simulink model "ColourTesting02_16_23"  (R2022a)
settings: Solver=VariableStepAuto  StartTime=0.0  StopTime=inf  RelTol=1e-3
model workspace (MAT data in the model file):
  SL_ROS_VariableLengthArrays_MaxSizes.CommonInfo.ArrayTruncateAction = 'EmitWarning'
  SL_ROS_VariableLengthArrays_MaxSizes.MsgTypeMap = containers.Map
  SL_ROS_VariableLengthArrays_MaxSizes.MsgTypeMap.serialization.keys = {'sensor_msgs/Image'}
  SL_ROS_VariableLengthArrays_MaxSizes.MsgTypeMap.serialization.values{1}(1).PropertyName = 'Data'
  SL_ROS_VariableLengthArrays_MaxSizes.MsgTypeMap.serialization.values{1}(1).DataType = 'uint8'
  SL_ROS_VariableLengthArrays_MaxSizes.MsgTypeMap.serialization.values{1}(1).MaxLength = 3686400
  SL_ROS_VariableLengthArrays_MaxSizes.MsgTypeMap.serialization.values{1}(2).PropertyName = 'Encoding'
  SL_ROS_VariableLengthArrays_MaxSizes.MsgTypeMap.serialization.values{1}(2).DataType = 'uint8'
  SL_ROS_VariableLengthArrays_MaxSizes.MsgTypeMap.serialization.values{1}(2).MaxLength = 128
  SL_ROS_VariableLengthArrays_MaxSizes.MsgTypeMap.serialization.uniformity = 0
  SL_ROS_VariableLengthArrays_MaxSizes.MsgTypeMap.serialization.keyType = 'char'
  SL_ROS_VariableLengthArrays_MaxSizes.MsgTypeMap.serialization.valueType = 'any'
undefined symbols (not defined in the file): coder, ros
libraries: robotlib x13
settings Model: SimulationMode=accelerator  Creator=ll  LastModifiedBy=ll

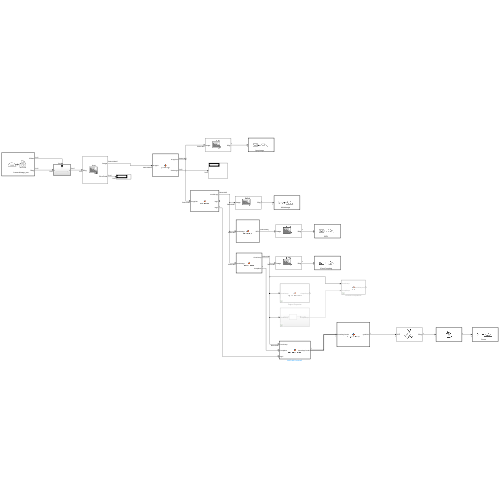
[thumbnail: Simulink's stored preview of the top-level diagram]
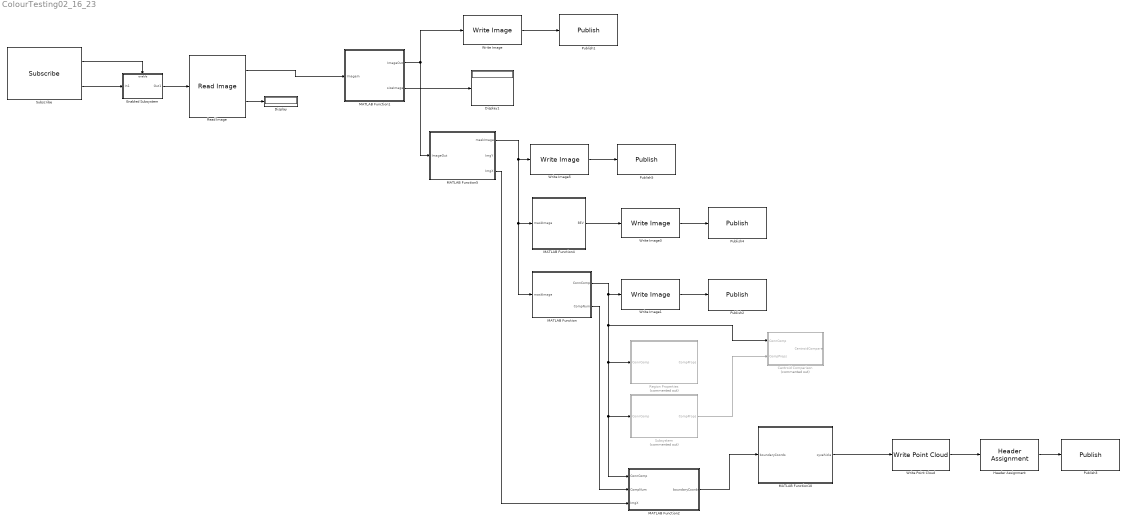
== system ColourTesting02_16_23 ==
  Centroid Comparison : MATLAB Function  Commented=on  TreatAsAtomicUnit=on
  Display : Display
  Display1 : Display
  Enabled Subsystem : Subsystem  TreatAsAtomicUnit=on
  Header Assignment : robotlib/Header Assignment  SetFrameID=on  FrameID=map  InsertTimeStamp=on  SetHeaderFieldName=Use the default Header field name  HeaderFieldName=Header
      settings: SourceProductBaseCode=RR
  MATLAB Function : MATLAB Function  TreatAsAtomicUnit=on
  MATLAB Function1 : MATLAB Function  TreatAsAtomicUnit=on
  MATLAB Function10 : MATLAB Function  TreatAsAtomicUnit=on
  MATLAB Function2 : MATLAB Function  TreatAsAtomicUnit=on
  MATLAB Function4 : MATLAB Function  TreatAsAtomicUnit=on
  MATLAB Function5 : MATLAB Function  TreatAsAtomicUnit=on
  Publish1 : robotlib/Publish  topicSource=Specify your own  topic=/grayimage  messageType=sensor_msgs/Image  legacyBusStruct=off  messageQueueLength=1
  Publish2 : robotlib/Publish  topicSource=Specify your own  topic=/ConnCompImg  messageType=sensor_msgs/Image  legacyBusStruct=off  messageQueueLength=1
  Publish3 : robotlib/Publish  topicSource=Specify your own  topic=/lanes  messageType=sensor_msgs/PointCloud2  legacyBusStruct=off  messageQueueLength=1
  Publish4 : robotlib/Publish  topicSource=Specify your own  topic=/BEV  messageType=sensor_msgs/Image  legacyBusStruct=off  messageQueueLength=1
  Publish5 : robotlib/Publish  topicSource=Specify your own  topic=/whiteimage  messageType=sensor_msgs/Image  legacyBusStruct=off  messageQueueLength=1
  Read Image : robotlib/Read Image  MaximumImageSize=[960, 1280]  ImageEncoding=bgr8  ShowAlphaOutput=off  ShowErrorCodeOutput=on  VariableSizeOutputs=off
      settings: SourceProductBaseCode=RR
  Region Properties : MATLAB Function  Commented=on  TreatAsAtomicUnit=on
  Subscribe : robotlib/Subscribe  topicSource=Select from ROS network  topic=/camera/image_raw  messageType=sensor_msgs/Image  SampleTime=-1  legacyBusStruct=off  messageQueueLength=1
  Subsystem : Subsystem  Commented=on
  Write Image{,1,3,5} (4 alike) : robotlib/Write Image  ImageEncoding=mono8  EncodingStruct=ros.msg.sensor_msgs.internal.ImageEncoding.info(coder.const('mono8'))  HasAlpha=off  messageType=sensor_msgs/Image
      settings: SourceProductBaseCode=RR
  Write Point Cloud : robotlib/Write Point Cloud  Encoding=none  HasRGB=false  HasAlpha=false  FieldNamesStruct=struct('x', 'single', 'y', 'single', 'z', 'single')  messageType=sensor_msgs/PointCloud2
      settings: SourceProductBaseCode=RR
  wires:
  Subscribe/2 -> Enabled Subsystem/1(In1)
  Enabled Subsystem/1(Out1) -> Read Image/1
  Subscribe/1 -> Enabled Subsystem/Enable
  Read Image/2 -> Display/1
  Read Image/1 -> MATLAB Function1/1(ImageIn)
  Write Image/1 -> Publish1/1
  MATLAB Function1/1(ImageOut) -> MATLAB Function5/1(ImageOut), Write Image/1
  MATLAB Function1/2(sizeImage) -> Display1/1
  MATLAB Function5/1(maskImage) -> MATLAB Function4/1(maskImage), MATLAB Function/1(maskImage), Write Image5/1
  Write Image5/1 -> Publish5/1
  MATLAB Function4/1(BEV) -> Write Image3/1
  Write Image3/1 -> Publish4/1
  MATLAB Function/1(ConnComp) -> Centroid Comparison/1(ConnComp), MATLAB Function2/1(ConnComp), Subsystem/1(ConnComp), Region Properties/1(ConnComp), Write Image1/1
  Write Image1/1 -> Publish2/1
  Subsystem/1(CompProps) -> Centroid Comparison/2(CompProps)
  MATLAB Function2/1(boundaryCoords) -> MATLAB Function10/1(boundaryCoords)
  MATLAB Function/2(CompNum) -> MATLAB Function2/2(CompNum)
  MATLAB Function5/3(ImgX) -> MATLAB Function2/3(ImgX)
  Header Assignment/1 -> Publish3/1
  Write Point Cloud/1 -> Header Assignment/1
  MATLAB Function10/1(xyvehicle) -> Write Point Cloud/1

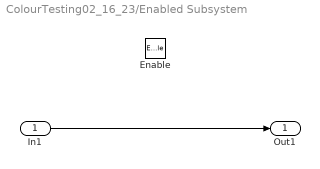
== system ColourTesting02_16_23/Enabled Subsystem ==
  In1 : Inport
  Enable : EnablePort
  Out1 : Outport
  wires:
  In1/1 -> Out1/1

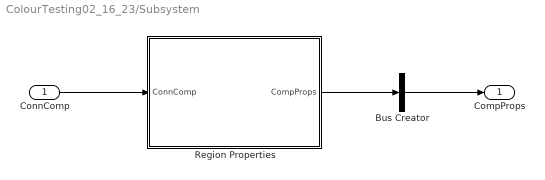
== system ColourTesting02_16_23/Subsystem ==
  ConnComp : Inport
  Bus Creator : BusCreator  Inputs=1
  Region Properties : MATLAB Function  TreatAsAtomicUnit=on
  CompProps : Outport
  wires:
  ConnComp/1 -> Region Properties/1(ConnComp)
  Region Properties/1(CompProps) -> Bus Creator/1
  Bus Creator/1 -> CompProps/1

== matlab function ColourTesting02_16_23/MATLAB Function1 ==
  data: ImageIn input; ImageOut output; sizeImage output
function [ImageOut,sizeImage] = grayImage(ImageIn)

sizeImage=size(ImageIn);

ImageOut=im2uint8(im2gray(ImageIn));

== matlab function ColourTesting02_16_23/MATLAB Function4 ==
  data: maskImage input; BEV output
function BEV = BEVimage(maskImage)
%Transform Road Image to Bird's-Eye-View Image
%Create a bird's-eye-view image from an image obtained by a front-facing 
% camera mounted on a vehicle. Display points within the bird's-eye view 
% using the vehicle and image coordinate systems.
%Define the camera intrinsics and create an object containing these intrinsics.
%focalLength = [309.4362 344.2161];
%focalLength=[274.769879268627	124.585825090253];
focalLength=[9.485122935354788e+02,9.419404214092846e+02];
%249.386359893401	113.313356588451
%principalPoint = [318.9034 257.5352];
%principalPoint = [618.652151593579	622.123926433697];
principalPoint = [5.819667727643726e+02,4.692273010971225e+02];
%617.370454615737	627.572919668628

%imageSize = [480 640];
imageSize = [960	1280];

%datasize=size(xyimageLeft);

camIntrinsics = cameraIntrinsics(focalLength,principalPoint,imageSize);

%Set the height of the camera to be about 2 meters above the ground. 
% Set the pitch of the camera to 14 degrees toward the ground.
 height = 1.85;
 pitch = 16.6;
% 
%Create an object containing the camera configuration.
sensor = monoCamera(camIntrinsics,height,'Pitch',pitch);
% 
% %Define the area in front of the camera that you want to transform into 
% a bird's-eye view. Set an area from 3 to 30 meters in front of the camera, 
% with 6 meters to either side of the camera.
distAhead = 5;
spaceToOneSide = 6;
bottomOffset = 0.5;
outView = [bottomOffset,distAhead,-spaceToOneSide,spaceToOneSide];

%Set the output image width to 250 pixels. Compute the output length 
% automatically from the width by setting the length to NaN.
outImageSize = [2879,1280];
%Create an object for performing bird's-eye-view transforms, using the 
% previously defined parameters.
birdsEye = birdsEyeView(sensor,outView,outImageSize);

BEV1 = transformImage(birdsEye,maskImage);
BEV = imresize(BEV1,[2500 1280]);

== matlab function ColourTesting02_16_23/Region Properties ==
  settings: updateMethod=CONTINUOUS
  data: ConnComp input; CompProps output
function CompProps = regionProperties(ConnComp)

CompProps = regionprops(ConnComp, 'all');

== matlab function ColourTesting02_16_23/MATLAB Function ==
  data: maskImage input; ConnComp output uint8; CompNum output
function [ConnComp,CompNum]= ConnComp(maskImage) 
initStrel = strel('diamond',3);
erodeImg = imerode(maskImage, initStrel);
ConnComp = bwareaopen(erodeImg , 2000);%remove components less that 2000 pixels

%use 8 connectivity to have accurate # of comp, we dont need to be
%filtering in this step
[CompLabels,CompNum] = bwlabel(ConnComp,8);

== matlab function ColourTesting02_16_23/MATLAB Function5 ==
  data: ImageOut input; maskImage output; ImgY output; ImgX output
function [maskImage,ImgY, ImgX]= whiteMask(ImageOut) 
[ImgY, ImgX, ColourLayers] = size(ImageOut);
maskImage1 = zeros(size(ImageOut,1),size(ImageOut,2));

% %----------------------Define thresholds for 'Hue'---------------------
 %channel1MinW = 200;
 %channel1MaxW = 255;
% %------------------Define thresholds for 'Saturation'------------------
% channel2MinW = 200;
% channel2MaxW = 255;
% %---------------------Define thresholds for 'Value'--------------------
% channel3MinW = 200;
% channel3MaxW = 255;

%-----------Create mask based on chosen histogram thresholds-----------

for i = 1:size(ImageOut,1)
    for j = 1:size(ImageOut,2)
        if ((ImageOut(i,j)>=249))
            maskImage1(i,j)  = 255;
        end
    end
end

maskImage = im2uint8(maskImage1);
 %maskImage=(ImageOut(:,:)>=channel1MinW)|(ImageOut(:,:)<=channel1MaxW);


%maskImage = imresize(maskImage1, [600 1280]);

== matlab function ColourTesting02_16_23/Centroid Comparison ==
  data: ConnComp input; CompProps input; CentroidCompare output
function CentroidCompare = fcn(ConnComp, CompProps)

allCompCentroids = vertcat(CompProps.Centroid);		% A 10 row by 2 column array of (x,y) centroid coordinates.
centroidsX = allCompCentroids(:, 1);			% Extract out the centroid x values into their own vector.
centroidsY = allCompCentroids(:, 2);

BinSize = 10;
BinNum = ImgX/BinSize;
BinStart=1;
Bin = 1;

for BinEnd=BinSize:BinSize:1280
WhiteX(Bin,1) = sum(ConnComp(:,BinStart:BinEnd-1),'all');
Bin = Bin+1;
BinStart=BinEnd;
end

plot(WhiteX)
axis([0 BinNum 0 max(WhiteX)])
%find local maximums because each peak has mulitple points so just maxs
%wont work
MinProm = 500;
LocalMaxima = islocalmax(WhiteX, "MinProminence",MinProm);
[maximaR, maximaC] = find(LocalMaxima==1);

%now that we have local max index, we compare to whiteX to get value and then we grab the two maxes from there. 
for k=1:1:size(maximaR)
LocalMaxValues(k,1) = WhiteX(maximaR(k),1);
end 

LaneMaxValues = maxk(LocalMaxValues,2);
[LaneMaxR(1), LaneMaxC(1)] = find(WhiteX==LaneMaxValues(1));
[LaneMaxR(2), LaneMaxC(2)] = find(WhiteX==LaneMaxValues(2));
%convert back to coord
CalcCenters = LaneMaxR(:)*BinSize;

%Comparing cetroids to white graph maxima to check if what we have are lane lines
WhitePtTolerance = BinSize + 7; %adding a little bit of extra tolerance because these aren't in bird's eye
CompInfo = zeros(CompNum, 2);
for i = 1:1:CompNum
    CompInfo (i,1) = centroidsX(i);
    CompInfo(i,2) = 0; %initalize to prevet false pos
    CentroidDifference1 = abs(CalcCenters(1)-centroidsX(i));
    CentroidDifference2 = abs(CalcCenters(2)-centroidsX(i));

    if (CentroidDifference1 <= WhitePtTolerance || CentroidDifference2 <= WhitePtTolerance)
        CompInfo(i,2) = 1; %true does match
    end 
end

== matlab function ColourTesting02_16_23/Subsystem/Region Properties ==
  settings: updateMethod=CONTINUOUS
  data: ConnComp input; CompProps output
function CompProps = regionProperties(ConnComp)

CompProps = regionprops(ConnComp, 'all');

== matlab function ColourTesting02_16_23/MATLAB Function2 ==
  data: ConnComp input; boundaryCoords output [..1280]; CompNum input; ImgX input
function boundaryCoords  = findBoundaries(ConnComp, CompNum, ImgX)
%CompProps = struct('centroid', 0);
%CompNum = max(CompLabels,[],'all','linear');
CompProps = regionprops(ConnComp, 'Centroid')
%ERROR: accessing field or property of nonscalar struct or object not supported
%for code generation in this context
%the following is a work around from https://stackoverflow.com/questions/72298202/how-to-solve-directly-accessing-field-or-property-of-nonscalar-struct-or-object

PropNums = numel(CompProps);
centroidPoints = coder.nullcopy(zeros(PropNums,2, "double"));
for idx = 1:PropNums
    centroidPoints(idx,1) = CompProps(idx).Centroid;
end

%allCompCentroids = vertcat(CompProps.Centroid);% A 10 row by 2 column array of (x,y) centroid coordinates.
%centroidsX = allCompCentroids(:, 1);% Extract out the centroid x values into their own vector.
%centroidsY = allCompCentroids(:, 2);


BinSize = 10;
BinNum = ImgX/BinSize;
BinStart=1;
Bin = 1;
WhiteX = zeros(BinNum,1);
for BinEnd=BinSize:BinSize:1280
WhiteX(Bin,1) = sum(ConnComp(:,BinStart:BinEnd-1),'all');
Bin = Bin+1;
BinStart=BinEnd;
end

plot(WhiteX)
axis([0 BinNum 0 max(WhiteX)])
%find local maximums because each peak has mulitple points so just maxs
%wont work
MinProm = 500;
LocalMaxima = islocalmax(WhiteX, "MinProminence",MinProm);
[maximaR, maximaC] = find(LocalMaxima==1);
LocalMaxValues=zeros(CompNum,2);
LaneMaxR=zeros(CompNum,2);
LaneMaxC=zeros(CompNum,2);
%now that we have local max index, we compare to whiteX to get value and then we grab the two maxes from there.
for k=1:1:numel(maximaR)
LocalMaxValues(k,1) = WhiteX(maximaR(k),1);
end

LaneMaxValues = maxk(LocalMaxValues,2);
[LaneMaxR(1), LaneMaxC(1)] = find(WhiteX==LaneMaxValues(1));
[LaneMaxR(2), LaneMaxC(2)] = find(WhiteX==LaneMaxValues(2));
%convert back to coord
CalcCenters = LaneMaxR(:)*BinSize;


%Comparing cetroids to white graph maxima to check if what we have are lane lines
WhitePtTolerance = BinSize + 7; %adding a little bit of extra tolerance because these aren't in bird's eye
CompInfo = zeros(CompNum, 2);
for i = 1:1:CompNum
    CompInfo (i,1) = centroidPoints(i,1);
    CompInfo(i,2) = 0; %initalize to prevet false pos
    CentroidDifference1 = abs(CalcCenters(1)-centroidPoints(i,1));
    CentroidDifference2 = abs(CalcCenters(2)-centroidPoints(i,2));

    if (CentroidDifference1 <= WhitePtTolerance || CentroidDifference2 <= WhitePtTolerance)
        CompInfo(i,2) = 1; %true does match
    end
end

%boundaryCoords = zeros(960,1280,CompNum);
    coder.varsize('CompBoundries',[960 1280], [1 0]);
for k = 1 : CompNum           % Loop through all comp.
    % Place the comp label number at the centroid of the blob.
    if(CompInfo(k,2)==1)
%text(centroidsX(k), centroidsY(k), num2str(k), 'FontSize', 14, 'FontWeight', 'Bold', 'HorizontalAlignment', 'center', 'VerticalAlignment', 'middle');
    CompBoundries = bwboundaries(ConnComp,8,'noholes');
    hold on;
    thisBoundary = CompBoundries{k}; % Get boundary for this component
    boundaryCoords = thisBoundary(:,:,k); % Column 2 is the columns, which is x % Column 1 is the rows, which is y
    %plot(x, y, 'r-', 'LineWidth', 3.5); % Plot boundary in red.
    end
end

== matlab function ColourTesting02_16_23/MATLAB Function10 ==
  data: boundaryCoords input; xyvehicle output
function xyvehicle  = image2distance(boundaryCoords)
%#codegen

%xyimageLeft(1,:)=xyimageLeft(1,:);
%xyimageRight(1,:)=xyimageRight(1,:);

%Transform Road Image to Bird's-Eye-View Image
%Create a bird's-eye-view image from an image obtained by a front-facing camera mounted on a vehicle. Display points within the bird's-eye view using the vehicle and image coordinate systems.
%Define the camera intrinsics and create an object containing these intrinsics.
%focalLength = [309.4362 344.2161];
%focalLength=[274.769879268627	124.585825090253];
focalLength=[950.730389523017	872.418095589972];
%249.386359893401	113.313356588451
%principalPoint = [318.9034 257.5352];
%principalPoint = [618.652151593579	622.123926433697];
principalPoint = [666.407201481039	199.198016715410];
%617.370454615737	627.572919668628

%imageSize = [480 640];
imageSize = [960	1280];
%datasize=size(xyimageLeft);

camIntrinsics = cameraIntrinsics(focalLength,principalPoint,imageSize);

%Set the height of the camera to be about 2 meters above the ground. Set the pitch of the camera to 14 degrees toward the ground.
 height = 1.85;
 pitch = 16.6;
% 
%Create an object containing the camera configuration.
sensor = monoCamera(camIntrinsics,height,'Pitch',pitch);
% 
% % %Define the area in front of the camera that you want to transform into a bird's-eye view. Set an area from 3 to 30 meters in front of the camera, with 6 meters to either side of the camera.
% distAhead = 30;
% spaceToOneSide = 6;
% bottomOffset = 3;
% outView = [bottomOffset,distAhead,-spaceToOneSide,spaceToOneSide];

% %Define the area in front of the camera that you want to transform into a bird's-eye view. Set an area from 3 to 30 meters in front of the camera, with 6 meters to either side of the camera.
distAhead = 5;
spaceToOneSide = 6;
bottomOffset = 1;
outView = [bottomOffset,distAhead,-spaceToOneSide,spaceToOneSide];

%Set the output image width to 250 pixels. Compute the output length automatically from the width by setting the length to NaN.
%outImageSize = [1024,250];
outImageSize = [2879,1280];


%Create an object for performing bird's-eye-view transforms, using the previously defined parameters.
birdsEye = birdsEyeView(sensor,outView,outImageSize);
%xyL=[xyimageLeft(1,:)'*dwidth,xyimageLeft(1,:)'*dheight];%
%xyL=imageToVehicle(birdsEye,xyimageLeft');
%xyR=[xyimageRight(1,:)'*dwidth,xyimageRight(1,:)'*dheight];%
%xyR=imageToVehicle(birdsEye,xyimageRight');

%xyR2=
xyLane=imageToVehicle(birdsEye,boundaryCoords');

%xyvehicleleft = single([xyL,zeros(length(xyL),1)]);
%xyvehicleright= single([xyR,zeros(length(xyR),1)]);
xyvehicle= single([xyLane,zeros(length(xyLane),1)]);
%datasizeL=size(xyvehicleleft);
%datasizeR=size(xyvehicleright);
datasize=size(xyvehicle);
